simulink model "pd_lq1"  (Simulink 4.00)
settings: Solver=ode45  StartTime=0.0  StopTime=100.0  RelTol=1e-3
values from neighbouring files (symbols this model uses):
  B = 0.1    [para_pdwithfriction.m]    (also in paradob.m)
  J = 0.005    [para_pdwithfriction.m]    (also in paradob.m)
  Kp = 0.6    [para_pdwithfriction.m]    (also in paradob.m)
  Kv = 0.01    [para_pdwithfriction.m]    (also in paradob.m)
  lqden = [1,-2.000029914714,1.00002921638403,0,0,0]    [para_pdwithfriction.m]    (also in paradob.m = [1.00000000000000,-1.99999255896952, 0.99999888907540,0,0,0])
  lqnum = [0.46520984850875,-1.38129465197227,0.89464551890550,0.95182605096981,-1.38845934950304,0.45807258302141]    [para_pdwithfriction.m]    (also in paradob.m = [4175.18064782253900,-12402.82692341595400,8044.365922430451)
  ts = 0.001    [para_pdwithfriction.m]    (also in paradob.m)
libraries: simulink3 x1
settings Model: LastModifiedBy=liuyuan1

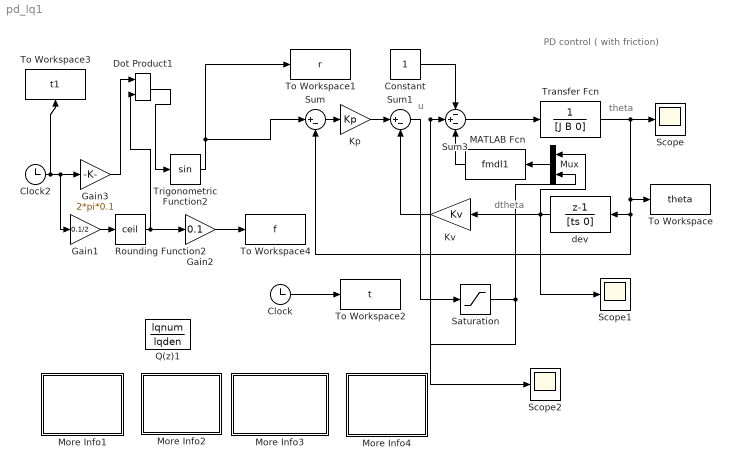
== system pd_lq1 ==
  note: theta
  note: dtheta
  note: u
  note: PD control ( with friction)
  " Kv" : Gain  Orientation=left  Gain=Kv  Multiplication=Element-wise(K.*u)  SaturateOnIntegerOverflow=on
  Clock : Clock
      settings: DisplayTime=off  Decimation=10
  Clock2 : Clock
      settings: Decimation=10
  Constant : Constant  Value=1
  Dot Product1 : simulink3/Math/Dot Product
  Gain1 : Gain  Gain=0.1/2  Multiplication=Element-wise(K.*u)  SaturateOnIntegerOverflow=on
  Gain2 : Gain  Gain=0.1  Multiplication=Element-wise(K.*u)  SaturateOnIntegerOverflow=on
  Gain3 : Gain  Gain=2*pi*0.1  Multiplication=Element-wise(K.*u)  SaturateOnIntegerOverflow=on
  "Kp " : Gain  Gain=Kp  Multiplication=Element-wise(K.*u)  SaturateOnIntegerOverflow=on
  MATLAB Fcn : MATLABFcn  Orientation=left  MATLABFcn=fmdl1  OutputDimensions=-1  OutputSignalType=auto  Output1D=on
      settings: AttributesFormatString=fmdl1
  More Info1 : Subsystem
      settings: OpenFcn=eval(['para_pdwithfriction']);  RTWFcnNameOpts=Auto  RTWFileNameOpts=Auto
      mask Display: disp('Double click\nhere for\nload parameters')
  More Info2 : Subsystem
      settings: OpenFcn=eval(['postpdwithfriction']);  RTWFcnNameOpts=Auto  RTWFileNameOpts=Auto
      mask Display: disp('Double click\nhere for plot')
  More Info3 : Subsystem
      settings: OpenFcn=eval(['test_freq']);  RTWFcnNameOpts=Auto  RTWFileNameOpts=Auto
      mask Display: disp('Double click\nhere for \ncompute frequency')
  More Info4 : Subsystem
      settings: OpenFcn=eval(['bode_plot']);  RTWFcnNameOpts=Auto  RTWFileNameOpts=Auto
      mask Display: disp('Double click\nhere for \ndraw bode')
  Mux : Mux  Orientation=left  Inputs=2
  Q(z)1 : DiscreteTransferFcn  Numerator=lqnum  Denominator=lqden  SampleTime=0.001  Realization=auto
      settings: RTWStateStorageClass=Auto
  Rounding Function2 : Rounding  Operator=ceil
  Saturation : Saturate  UpperLimit=10  LowerLimit=-10  LinearizeAsGain=on
  Scope : Scope
      settings: TimeRange=auto  YMin=-2.75  YMax=-0.75  SaveToWorkspace=off  LimitDataPoints=on  MaxDataPoints=6000
  Scope1 : Scope
      settings: TimeRange=auto  YMin=-40  YMax=60  SaveToWorkspace=off  SaveName=ScopeData2  LimitDataPoints=on  MaxDataPoints=6000
  Scope2 : Scope
      settings: TimeRange=auto  YMin=-7.5  YMax=15  SaveToWorkspace=off  SaveName=ScopeData  LimitDataPoints=on  MaxDataPoints=6000
  Sum : Sum  Inputs=|+-  SaturateOnIntegerOverflow=on
  Sum1 : Sum  Inputs=|+-  SaturateOnIntegerOverflow=on
  Sum3 : Sum  Inputs=-+-  SaturateOnIntegerOverflow=on
  To Workspace : ToWorkspace  VariableName=theta  SampleTime=-1  SaveFormat=Array
  To Workspace1 : ToWorkspace  VariableName=r  SampleTime=-1  SaveFormat=Array
  To Workspace2 : ToWorkspace  VariableName=t  SampleTime=-1  SaveFormat=Array
  To Workspace3 : ToWorkspace  VariableName=t1  SampleTime=-1  SaveFormat=Array
      settings: Orientation=up
  To Workspace4 : ToWorkspace  VariableName=f  SampleTime=-1  SaveFormat=Array
  Transfer Fcn : TransferFcn  Numerator=[0 0 1]  Denominator=[J B 0]  AbsoluteTolerance=auto  Realization=auto
  Trigonometric Function2 : Trigonometry  Operator=sin  OutputSignalType=auto
  dev : DiscreteTransferFcn  Orientation=left  Numerator=[1 -1]  Denominator=[ts 0]  SampleTime=0.001  Realization=auto
      settings: RTWStateStorageClass=Auto
  wires:
  Sum/1 -> "Kp "/1
  "Kp "/1 -> Sum1/1
  Transfer Fcn/1 -> Scope/1, dev/1, Sum/2, To Workspace/1
  " Kv"/1 -> Sum1/2
  dev/1 -> " Kv"/1, Scope1/1, Mux/1
  Sum3/1 -> Transfer Fcn/1
  Clock/1 -> To Workspace2/1
  Mux/1 -> MATLAB Fcn/1
  Sum1/1 -> Saturation/1
  MATLAB Fcn/1 -> Sum3/3
  Trigonometric Function2/1 -> To Workspace1/1, Sum/1
  Clock2/1 -> Gain3/1, Gain1/1, To Workspace3/1
  Gain1/1 -> Rounding Function2/1
  Gain3/1 -> Dot Product1/1
  Dot Product1/1 -> Trigonometric Function2/1
  Rounding Function2/1 -> Gain2/1, Dot Product1/2
  Gain2/1 -> To Workspace4/1
  Saturation/1 -> Mux/2, Scope2/1, Sum3/2
  Constant/1 -> Sum3/1

== system pd_lq1/More Info1 ==

== system pd_lq1/More Info2 ==

== system pd_lq1/More Info3 ==

== system pd_lq1/More Info4 ==
